simulink model "MyModel_Open_v1_r2016b"  (R2016b)
settings: Solver=ode23tb  StartTime=0.0  StopTime=0.3  MaxStep=1e-6  RelTol=1e-4
InitFcn:
  | Udc1 = 200;
  | Udc2 = 200;
  | tpwm = 1e-4;
  | ratio = Udc1/Udc2;
  | Td = 2e-6;
  | Kp_current = 3;
  | Ki_current = 120;
libraries: powerlib x31, powerlib_meascontrol x24, powerlib_extras x5, simulink_extras x2, simulink x2
(part 1 of 2)
settings Model: Creator=chenhao  LastModifiedBy=chenhao
settings SFSimCC: SimUseLocalCustomCode=on
settings RTWCC: RTWUseLocalCustomCode=on

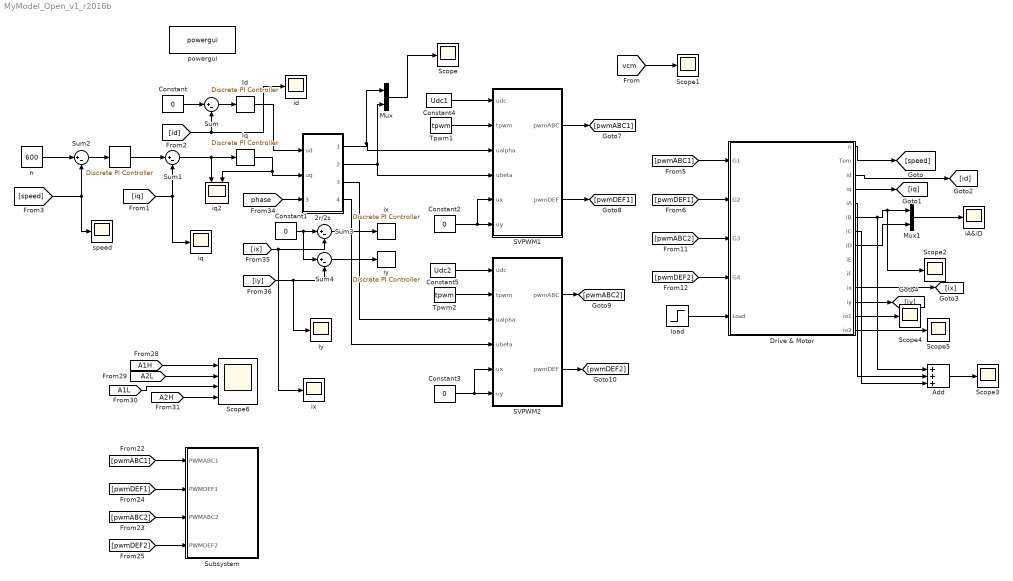
== system MyModel_Open_v1_r2016b ==
  "    " : powerlib_extras/Discrete  Control Blocks/Discrete PI Controller  Kp=1  Ki=100  Par_Limits=[50 -50]  Init=0  Ts=tpwm
  " Id" : powerlib_extras/Discrete  Control Blocks/Discrete PI Controller  Kp=Kp_current  Ki=Ki_current  Par_Limits=[300 -300]  Init=0  Ts=tpwm
  " Iq" : powerlib_extras/Discrete  Control Blocks/Discrete PI Controller  Kp=Kp_current  Ki=Ki_current  Par_Limits=[300 -300]  Init=0  Ts=tpwm
  " ix" : powerlib_extras/Discrete  Control Blocks/Discrete PI Controller  Kp=10  Ki=100  Par_Limits=[300 -300]  Init=0  Ts=tpwm
  " iy" : powerlib_extras/Discrete  Control Blocks/Discrete PI Controller  Kp=10  Ki=100  Par_Limits=[300 -300]  Init=0  Ts=tpwm
  2r/2s : Subsystem
  Add : Sum  Inputs=3
  Constant{,1..3} (4 alike) : Constant  Value=0
  Constant4 : Constant  Value=Udc1
  Constant5 : Constant  Value=Udc2
  Drive & Motor : Subsystem
  Mux : Mux  Inputs=2
  Mux1 : Mux  Inputs=2
  SVPWM1 : Subsystem
  SVPWM2 : Subsystem
  Scope{,1..5} (6 alike) : Scope
  Scope6 : Scope  NumInputPorts=4
  Subsystem : Subsystem
  Sum{,1..4} (5 alike) : Sum  Inputs=|+-
  Tpwm1 : Constant  Value=tpwm
  Tpwm2 : Constant  Value=tpwm
  "iA&iD " : Scope
  "id " : Scope
  iq : Scope
  iq2 : Scope  NumInputPorts=2
  ix : Scope
  iy : Scope
  load : Step  Time=0  After=15  SampleTime=0
  n : Constant  Value=600
  powergui : powerlib/powergui  Priority=1  SimulationMode=Continuous  SampleTime=1E-6  frequency=60  Iterations=50  frequencyindice=0  Pbase=100e6  ErrMax=1e-4  UnitsV=kV  UnitsW=MW  buscounter=0  FunctionMessages=off  echomessages=off  EnableUseOfTLC=off  CurrentSourceSwitches=off  DisableSnubberDevices=off  DisableRonSwitches=off  DisableVfSwitches=off  DisplayEquations=off  SolverType=Tustin/Backward Euler (TBE)  Interpol=off  ExternalGateDelay=off  methode=off  Ts=100  x0status=blocks  SPID=off  SwTol=0  HookPort=off  RestoreLinks=warning  ResistiveCurrentMeasurement=off  Frange=[0:2:500]  Ylog=off  Xlog=on  ShowGrid=off  save=off  variable=ZData  structure=IA  ZoomFFT=off  StartTime=0.2  cycles=3  DisplayStyle=1  fundamental=50  FreqAxis=on  MaxFrequency=1000  frequencyindicesteady=1  RmsSteady=1  display=off
  "speed " : Scope
  wires:
  2r/2s/2(ubeta1) -> SVPWM1/4(ubeta), Mux/2
  Mux/1 -> Scope/1
  Tpwm1/1 -> SVPWM1/2(tpwm)
  load/1 -> Drive & Motor/5(Load)
  [iy] -> iy/1, Sum4/2
  [iq] -> iq/1, Sum1/2
  Sum3/1 -> " ix"/1
  Constant4/1 -> SVPWM1/1(udc)
  Sum2/1 -> "    "/1
  2r/2s/1(ualfa1) -> SVPWM1/3(ualpha), Mux/1
  Sum1/1 -> iq2/1, " Iq"/1
  [speed] -> "speed "/1, Sum2/2
  Sum4/1 -> " iy"/1
  n/1 -> Sum2/1
  [ix] -> ix/1, Sum3/2
  " Id"/1 -> 2r/2s/1(ud)
  [phase] -> 2r/2s/3(theta)
  " Iq"/1 -> iq2/2, 2r/2s/2(uq)
  Sum/1 -> " Id"/1
  Constant1/1 -> Sum4/1, Sum3/1
  "    "/1 -> Sum1/1
  [id] -> "id "/1, Sum/2
  Constant/1 -> Sum/1
  Drive & Motor/1(n) -> [speed]
  Drive & Motor/4(iq) -> [iq]
  Drive & Motor/3(id) -> [id]
  Drive & Motor/11(ix) -> [ix]
  Drive & Motor/12(iy) -> [iy]
  Drive & Motor/5(iA) -> Add/1, Scope2/1, Mux1/1
  Drive & Motor/8(iD) -> Mux1/2
  Mux1/1 -> "iA&iD "/1
  Constant5/1 -> SVPWM2/1(udc)
  Tpwm2/1 -> SVPWM2/2(tpwm)
  2r/2s/3(ualfa2) -> SVPWM2/3(ualpha)
  2r/2s/4(ubeta2) -> SVPWM2/4(ubeta)
  Constant2/1 -> SVPWM1/5(ux), SVPWM1/6(uy)
  Constant3/1 -> SVPWM2/6(uy), SVPWM2/5(ux)
  SVPWM1/2(pwmDEF) -> [pwmDEF1]
  SVPWM2/1(pwmABC) -> [pwmABC2]
  SVPWM1/1(pwmABC) -> [pwmABC1]
  SVPWM2/2(pwmDEF) -> [pwmDEF2]
  [pwmABC1] -> Drive & Motor/1(G1)
  [pwmDEF1] -> Drive & Motor/2(G2)
  [pwmABC2] -> Drive & Motor/3(G3)
  [pwmDEF2] -> Drive & Motor/4(G4)
  [vcm] -> Scope1/1
  [A1L] -> Scope6/3
  [A1H] -> Scope6/1
  [pwmABC1] -> Subsystem/1(PWMABC1)
  [A2L] -> Scope6/2
  [A2H] -> Scope6/4
  [pwmDEF1] -> Subsystem/2(PWMDEF1)
  [pwmABC2] -> Subsystem/3(PWMABC2)
  [pwmDEF2] -> Subsystem/4(PWMDEF2)
  Drive & Motor/6(iB) -> Add/2
  Drive & Motor/7(iC) -> Add/3
  Add/1 -> Scope3/1
  Drive & Motor/13(io1) -> Scope4/1
  Drive & Motor/14(io2) -> Scope5/1

== system MyModel_Open_v1_r2016b/2r//2s ==
  ud : Inport
  uq : Inport  Port=2
  theta : Inport  Port=3
  Fcn : Fcn  Expr=u(1)*cos(u(3))-u(2)*sin(u(3))
  Fcn1 : Fcn  Expr=u(1)*sin(u(3))+u(2)*cos(u(3))
  Gain : Gain  Gain=ratio /(ratio + 1)
  Gain1 : Gain  Gain=ratio /(ratio + 1)
  Gain2 : Gain  Gain=-1 /(ratio + 1)
  Gain3 : Gain  Gain=-1 /(ratio + 1)
  Mux1 : Mux  Inputs=3
  ualfa1 : Outport
  ubeta1 : Outport  Port=2
  ualfa2 : Outport  Port=3
  ubeta2 : Outport  Port=4
  wires:
  theta/1 -> Mux1/3
  uq/1 -> Mux1/2
  ud/1 -> Mux1/1
  Mux1/1 -> Fcn1/1, Fcn/1
  Fcn/1 -> Gain2/1, Gain/1
  Gain/1 -> ualfa1/1
  Gain1/1 -> ubeta1/1
  Fcn1/1 -> Gain3/1, Gain1/1
  Gain2/1 -> ualfa2/1
  Gain3/1 -> ubeta2/1

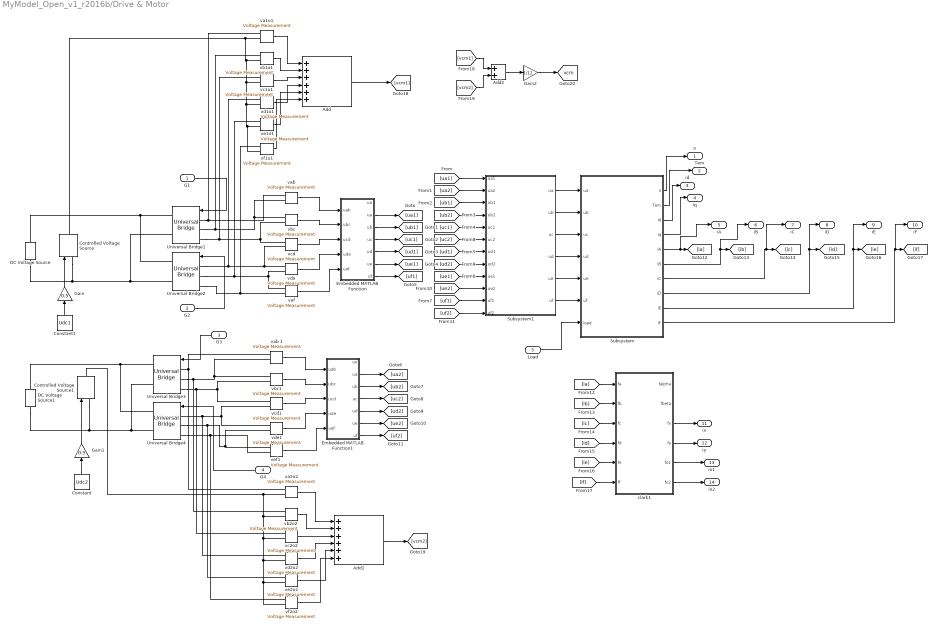
== system MyModel_Open_v1_r2016b/Drive & Motor ==
  G1 : Inport
  G2 : Inport  Port=2
  G3 : Inport  Port=3
  G4 : Inport  Port=4
  Load : Inport  Port=5
  Add : Sum  Inputs=++++++
  Add1 : Sum  Inputs=++++++
  Add2 : Sum
  Constant : Constant  Value=Udc2
  Constant1 : Constant  Value=Udc1
  Controlled Voltage Source : powerlib/Electrical Sources/Controlled Voltage Source  Initialize=on  Source_Type=AC  Amplitude=0  Phase=0  Frequency=0  Measurements=None
  Controlled Voltage Source1 : powerlib/Electrical Sources/Controlled Voltage Source  Initialize=on  Source_Type=AC  Amplitude=0  Phase=0  Frequency=0  Measurements=None
  DC Voltage Source : powerlib/Electrical Sources/DC Voltage Source  Amplitude=Udc1  Measurements=Voltage
  DC Voltage Source1 : powerlib/Electrical Sources/DC Voltage Source  Amplitude=Udc2  Measurements=Voltage
  Embedded MATLAB Function : MATLAB Function  TreatAsAtomicUnit=on
  Embedded MATLAB Function1 : MATLAB Function  TreatAsAtomicUnit=on
  Gain : Gain  Gain=0.5
  Gain1 : Gain  Gain=0.5
  Gain2 : Gain  Gain=1/12
  Subsystem : Subsystem
  Subsystem1 : Subsystem
  Universal Bridge{1..4} (4 alike) : powerlib/Power Electronics/Universal Bridge  Arms=3  SnubberResistance=1e5  SnubberCapacitance=inf  Device=IGBT / Diodes  Ron=1e-3  Lon=0  ForwardVoltages="[  0  0  ]"  ForwardVoltage=0  GTOparameters=[ 10e-6 , 20e-6 ]  IGBTparameters=[ 0 , 0 ]  Measurements=None  Measurements_2=None  converterType=Rectifier
  clark1 : MATLAB Function  TreatAsAtomicUnit=on
  va1o1 : powerlib/Measurements/Voltage Measurement  PhasorSimulation=off  OutputType=Complex  PSBequivalent=0
  va2o2 : powerlib/Measurements/Voltage Measurement  PhasorSimulation=off  OutputType=Complex  PSBequivalent=0
  "vab " : powerlib/Measurements/Voltage Measurement  PhasorSimulation=off  OutputType=Complex  PSBequivalent=0
  vab 1 : powerlib/Measurements/Voltage Measurement  PhasorSimulation=off  OutputType=Complex  PSBequivalent=0
  vb1o1 : powerlib/Measurements/Voltage Measurement  PhasorSimulation=off  OutputType=Complex  PSBequivalent=0
  vb2o2 : powerlib/Measurements/Voltage Measurement  PhasorSimulation=off  OutputType=Complex  PSBequivalent=0
  vbc : powerlib/Measurements/Voltage Measurement  PhasorSimulation=off  OutputType=Complex  PSBequivalent=0
  vbc1 : powerlib/Measurements/Voltage Measurement  PhasorSimulation=off  OutputType=Complex  PSBequivalent=0
  vc1o1 : powerlib/Measurements/Voltage Measurement  PhasorSimulation=off  OutputType=Complex  PSBequivalent=0
  vc2o2 : powerlib/Measurements/Voltage Measurement  PhasorSimulation=off  OutputType=Complex  PSBequivalent=0
  vcd : powerlib/Measurements/Voltage Measurement  PhasorSimulation=off  OutputType=Complex  PSBequivalent=0
  vcd1 : powerlib/Measurements/Voltage Measurement  PhasorSimulation=off  OutputType=Complex  PSBequivalent=0
  vd1o1 : powerlib/Measurements/Voltage Measurement  PhasorSimulation=off  OutputType=Complex  PSBequivalent=0
  vd2o2 : powerlib/Measurements/Voltage Measurement  PhasorSimulation=off  OutputType=Complex  PSBequivalent=0
  vde : powerlib/Measurements/Voltage Measurement  PhasorSimulation=off  OutputType=Complex  PSBequivalent=0
  vde1 : powerlib/Measurements/Voltage Measurement  PhasorSimulation=off  OutputType=Complex  PSBequivalent=0
  ve1o1 : powerlib/Measurements/Voltage Measurement  PhasorSimulation=off  OutputType=Complex  PSBequivalent=0
  ve2o2 : powerlib/Measurements/Voltage Measurement  PhasorSimulation=off  OutputType=Complex  PSBequivalent=0
  vef : powerlib/Measurements/Voltage Measurement  PhasorSimulation=off  OutputType=Complex  PSBequivalent=0
  vef1 : powerlib/Measurements/Voltage Measurement  PhasorSimulation=off  OutputType=Complex  PSBequivalent=0
  vf1o1 : powerlib/Measurements/Voltage Measurement  PhasorSimulation=off  OutputType=Complex  PSBequivalent=0
  vf2o2 : powerlib/Measurements/Voltage Measurement  PhasorSimulation=off  OutputType=Complex  PSBequivalent=0
  n : Outport
  Tem : Outport  Port=2
  id : Outport  Port=3
  iq : Outport  Port=4
  iA : Outport  Port=5
  iB : Outport  Port=6
  iC : Outport  Port=7
  iD : Outport  Port=8
  iE : Outport  Port=9
  iF : Outport  Port=10
  ix : Outport  Port=11
  iy : Outport  Port=12
  io1 : Outport  Port=13
  io2 : Outport  Port=14
  tag scope: vcm=global
  wires:
  G1/1 -> Universal Bridge1/1
  G2/1 -> Universal Bridge2/1
  G3/1 -> Universal Bridge3/1
  G4/1 -> Universal Bridge4/1
  vef/1 -> Embedded MATLAB Function/5(uef)
  vde/1 -> Embedded MATLAB Function/4(ude)
  "vab "/1 -> Embedded MATLAB Function/1(uab)
  vcd/1 -> Embedded MATLAB Function/3(ucd)
  vbc/1 -> Embedded MATLAB Function/2(ubc)
  Embedded MATLAB Function/2(ua) -> [ua1]
  Embedded MATLAB Function/3(ub) -> [ub1]
  Embedded MATLAB Function/4(uc) -> [uc1]
  Embedded MATLAB Function/5(ud) -> [ud1]
  Embedded MATLAB Function/6(ue) -> [ue1]
  Embedded MATLAB Function/7(uf) -> [uf1]
  Embedded MATLAB Function1/2(ua) -> [ua2]
  Embedded MATLAB Function1/3(ub) -> [ub2]
  Embedded MATLAB Function1/4(uc) -> [uc2]
  Embedded MATLAB Function1/5(ud) -> [ud2]
  Embedded MATLAB Function1/6(ue) -> [ue2]
  Embedded MATLAB Function1/7(uf) -> [uf2]
  vab 1/1 -> Embedded MATLAB Function1/1(uab)
  vbc1/1 -> Embedded MATLAB Function1/2(ubc)
  vcd1/1 -> Embedded MATLAB Function1/3(ucd)
  vde1/1 -> Embedded MATLAB Function1/4(ude)
  vef1/1 -> Embedded MATLAB Function1/5(uef)
  [ua1] -> Subsystem1/1(ua1)
  [ua2] -> Subsystem1/2(ua2)
  [ub1] -> Subsystem1/3(ub1)
  [ub2] -> Subsystem1/4(ub2)
  [uc1] -> Subsystem1/5(uc1)
  [uc2] -> Subsystem1/6(uc2)
  [ud1] -> Subsystem1/7(ud1)
  [ud2] -> Subsystem1/8(ud2)
  [ue1] -> Subsystem1/9(ue1)
  [ue2] -> Subsystem1/10(ue2)
  [uf1] -> Subsystem1/11(uf1)
  [uf2] -> Subsystem1/12(uf2)
  Subsystem1/1(ua) -> Subsystem/1(ua)
  Subsystem1/2(ub) -> Subsystem/2(ub)
  Subsystem1/3(uc) -> Subsystem/3(uc)
  Subsystem1/4(ud) -> Subsystem/4(ud)
  Subsystem1/5(ue) -> Subsystem/5(ue)
  Subsystem1/6(uf) -> Subsystem/6(uf)
  Load/1 -> Subsystem/7(load)
  Subsystem/1(n) -> n/1
  Subsystem/2(Tem) -> Tem/1
  Subsystem/3(id) -> id/1
  Subsystem/4(iq) -> iq/1
  Subsystem/5(iA) -> iA/1, [ia]
  Subsystem/6(iB) -> iB/1, [ib]
  Subsystem/7(iC) -> iC/1, [ic]
  Subsystem/8(iD) -> iD/1, [id]
  Subsystem/9(iE) -> iE/1, [ie]
  Subsystem/10(iF) -> iF/1, [if]
  [ia] -> clark1/1(fa)
  [ib] -> clark1/2(fb)
  [ic] -> clark1/3(fc)
  [id] -> clark1/4(fd)
  [ie] -> clark1/5(fe)
  [if] -> clark1/6(ff)
  clark1/3(fx) -> ix/1
  clark1/4(fy) -> iy/1
  Gain/1 -> Controlled Voltage Source/1
  Gain1/1 -> Controlled Voltage Source1/1
  va1o1/1 -> Add/1
  vb1o1/1 -> Add/2
  vc1o1/1 -> Add/3
  vd1o1/1 -> Add/4
  ve1o1/1 -> Add/5
  vf1o1/1 -> Add/6
  Add/1 -> [vcm1]
  va2o2/1 -> Add1/1
  vb2o2/1 -> Add1/2
  vc2o2/1 -> Add1/3
  vd2o2/1 -> Add1/4
  ve2o2/1 -> Add1/5
  vf2o2/1 -> Add1/6
  Add1/1 -> [vcm2]
  [vcm1] -> Add2/1
  [vcm2] -> Add2/2
  Add2/1 -> Gain2/1
  Gain2/1 -> [vcm]
  Constant/1 -> Gain1/1
  Constant1/1 -> Gain/1
  clark1/5(fo1) -> io1/1
  clark1/6(fo2) -> io2/1
  connections:
  vde1/LConn1 -- vcd1/LConn2 -- vd2o2/LConn1 -- Universal Bridge4/LConn1
  vde/LConn1 -- vd1o1/LConn1 -- Universal Bridge2/LConn1 -- vcd/LConn2
  vef1/LConn2 -- Universal Bridge4/LConn3 -- vf2o2/LConn1
  Universal Bridge1/RConn2 -- DC Voltage Source/LConn1 -- Controlled Voltage Source/LConn1 -- Universal Bridge2/RConn2
  DC Voltage Source/RConn1 -- Universal Bridge2/RConn1 -- Universal Bridge1/RConn1
  Universal Bridge3/LConn1 -- vab 1/LConn1 -- va2o2/LConn1
  vbc/LConn1 -- vb1o1/LConn1 -- Universal Bridge1/LConn2 -- "vab "/LConn2
  vbc1/LConn1 -- vb2o2/LConn1 -- Universal Bridge3/LConn2 -- vab 1/LConn2
  vcd/LConn1 -- vc1o1/LConn1 -- Universal Bridge1/LConn3 -- vbc/LConn2
  vbc1/LConn2 -- vc2o2/LConn1 -- Universal Bridge3/LConn3 -- vcd1/LConn1
  Universal Bridge3/RConn1 -- DC Voltage Source1/RConn1 -- Universal Bridge4/RConn1
  Universal Bridge3/RConn2 -- DC Voltage Source1/LConn1 -- Controlled Voltage Source1/LConn1 -- Universal Bridge4/RConn2
  vef1/LConn1 -- ve2o2/LConn1 -- Universal Bridge4/LConn2 -- vde1/LConn2
  Universal Bridge1/LConn1 -- "vab "/LConn1 -- va1o1/LConn1
  vef/LConn1 -- ve1o1/LConn1 -- Universal Bridge2/LConn2 -- vde/LConn2
  Universal Bridge2/LConn3 -- vf1o1/LConn1 -- vef/LConn2
  va1o1/LConn2 -- vf1o1/LConn2 -- ve1o1/LConn2 -- vd1o1/LConn2 -- vc1o1/LConn2 -- vb1o1/LConn2 -- Controlled Voltage Source/RConn1
  va2o2/LConn2 -- vf2o2/LConn2 -- ve2o2/LConn2 -- vd2o2/LConn2 -- vc2o2/LConn2 -- vb2o2/LConn2 -- Controlled Voltage Source1/RConn1

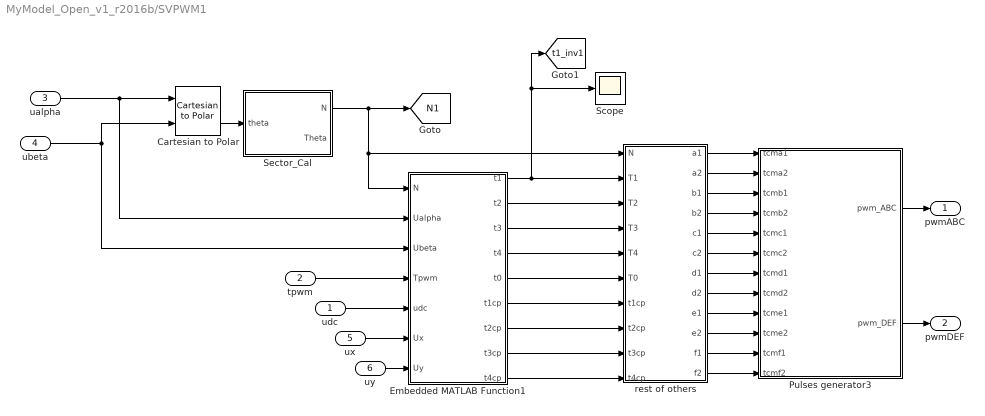
== system MyModel_Open_v1_r2016b/SVPWM1 ==
  udc : Inport
  tpwm : Inport  Port=2
  ualpha : Inport  Port=3
  ubeta : Inport  Port=4
  ux : Inport  Port=5
  uy : Inport  Port=6
  Cartesian to Polar : simulink_extras/Transformations/Cartesian to Polar
  Embedded MATLAB Function1 : MATLAB Function  TreatAsAtomicUnit=on
  Pulses generator3 : Subsystem
  Scope : Scope
  Sector_Cal : Subsystem
  rest of others : MATLAB Function  TreatAsAtomicUnit=on
  pwmABC : Outport
  pwmDEF : Outport  Port=2
  tag scope: N1=global, t1_inv1=global
  wires:
  tpwm/1 -> Embedded MATLAB Function1/4(Tpwm)
  ubeta/1 -> Cartesian to Polar/2, Embedded MATLAB Function1/3(Ubeta)
  ualpha/1 -> Cartesian to Polar/1, Embedded MATLAB Function1/2(Ualpha)
  ux/1 -> Embedded MATLAB Function1/6(Ux)
  uy/1 -> Embedded MATLAB Function1/7(Uy)
  udc/1 -> Embedded MATLAB Function1/5(udc)
  rest of others/12(f2) -> Pulses generator3/12(tcmf2)
  rest of others/11(f1) -> Pulses generator3/11(tcmf1)
  rest of others/9(e1) -> Pulses generator3/9(tcme1)
  rest of others/8(d2) -> Pulses generator3/8(tcmd2)
  rest of others/10(e2) -> Pulses generator3/10(tcme2)
  rest of others/2(a2) -> Pulses generator3/2(tcma2)
  rest of others/6(c2) -> Pulses generator3/6(tcmc2)
  rest of others/4(b2) -> Pulses generator3/4(tcmb2)
  rest of others/5(c1) -> Pulses generator3/5(tcmc1)
  rest of others/7(d1) -> Pulses generator3/7(tcmd1)
  rest of others/3(b1) -> Pulses generator3/3(tcmb1)
  rest of others/1(a1) -> Pulses generator3/1(tcma1)
  Embedded MATLAB Function1/1(t1) -> [t1_inv1], Scope/1, rest of others/2(T1)
  Embedded MATLAB Function1/2(t2) -> rest of others/3(T2)
  Embedded MATLAB Function1/3(t3) -> rest of others/4(T3)
  Embedded MATLAB Function1/4(t4) -> rest of others/5(T4)
  Embedded MATLAB Function1/5(t0) -> rest of others/6(T0)
  Embedded MATLAB Function1/6(t1cp) -> rest of others/7(t1cp)
  Embedded MATLAB Function1/7(t2cp) -> rest of others/8(t2cp)
  Embedded MATLAB Function1/8(t3cp) -> rest of others/9(t3cp)
  Embedded MATLAB Function1/9(t4cp) -> rest of others/10(t4cp)
  Cartesian to Polar/2 -> Sector_Cal/1(theta)
  Sector_Cal/1(N) -> [N1], rest of others/1(N), Embedded MATLAB Function1/1(N)
  Pulses generator3/1(pwm_ABC) -> pwmABC/1
  Pulses generator3/2(pwm_DEF) -> pwmDEF/1

== system MyModel_Open_v1_r2016b/SVPWM2 ==
  udc : Inport
  tpwm : Inport  Port=2
  ualpha : Inport  Port=3
  ubeta : Inport  Port=4
  ux : Inport  Port=5
  uy : Inport  Port=6
  Cartesian to Polar : simulink_extras/Transformations/Cartesian to Polar
  Embedded MATLAB Function1 : MATLAB Function  TreatAsAtomicUnit=on
  Pulses generator3 : Subsystem
  Scope : Scope
  Sector_Cal : Subsystem
  rest of others : MATLAB Function  TreatAsAtomicUnit=on
  pwmABC : Outport
  pwmDEF : Outport  Port=2
  tag scope: N2=global, t1_inv2=global
  wires:
  Pulses generator3/2(pwm_DEF) -> pwmDEF/1
  Pulses generator3/1(pwm_ABC) -> pwmABC/1
  Sector_Cal/1(N) -> [N2], Embedded MATLAB Function1/1(N), rest of others/1(N)
  Cartesian to Polar/2 -> Sector_Cal/1(theta)
  Embedded MATLAB Function1/9(t4cp) -> rest of others/10(t4cp)
  Embedded MATLAB Function1/8(t3cp) -> rest of others/9(t3cp)
  Embedded MATLAB Function1/7(t2cp) -> rest of others/8(t2cp)
  Embedded MATLAB Function1/6(t1cp) -> rest of others/7(t1cp)
  Embedded MATLAB Function1/5(t0) -> rest of others/6(T0)
  Embedded MATLAB Function1/4(t4) -> rest of others/5(T4)
  Embedded MATLAB Function1/3(t3) -> rest of others/4(T3)
  Embedded MATLAB Function1/2(t2) -> rest of others/3(T2)
  Embedded MATLAB Function1/1(t1) -> rest of others/2(T1), [t1_inv2], Scope/1
  rest of others/1(a1) -> Pulses generator3/1(tcma1)
  rest of others/3(b1) -> Pulses generator3/3(tcmb1)
  rest of others/7(d1) -> Pulses generator3/7(tcmd1)
  rest of others/5(c1) -> Pulses generator3/5(tcmc1)
  rest of others/4(b2) -> Pulses generator3/4(tcmb2)
  rest of others/6(c2) -> Pulses generator3/6(tcmc2)
  rest of others/2(a2) -> Pulses generator3/2(tcma2)
  rest of others/10(e2) -> Pulses generator3/10(tcme2)
  rest of others/8(d2) -> Pulses generator3/8(tcmd2)
  rest of others/9(e1) -> Pulses generator3/9(tcme1)
  rest of others/11(f1) -> Pulses generator3/11(tcmf1)
  rest of others/12(f2) -> Pulses generator3/12(tcmf2)
  udc/1 -> Embedded MATLAB Function1/5(udc)
  uy/1 -> Embedded MATLAB Function1/7(Uy)
  ux/1 -> Embedded MATLAB Function1/6(Ux)
  ualpha/1 -> Embedded MATLAB Function1/2(Ualpha), Cartesian to Polar/1
  ubeta/1 -> Embedded MATLAB Function1/3(Ubeta), Cartesian to Polar/2
  tpwm/1 -> Embedded MATLAB Function1/4(Tpwm)

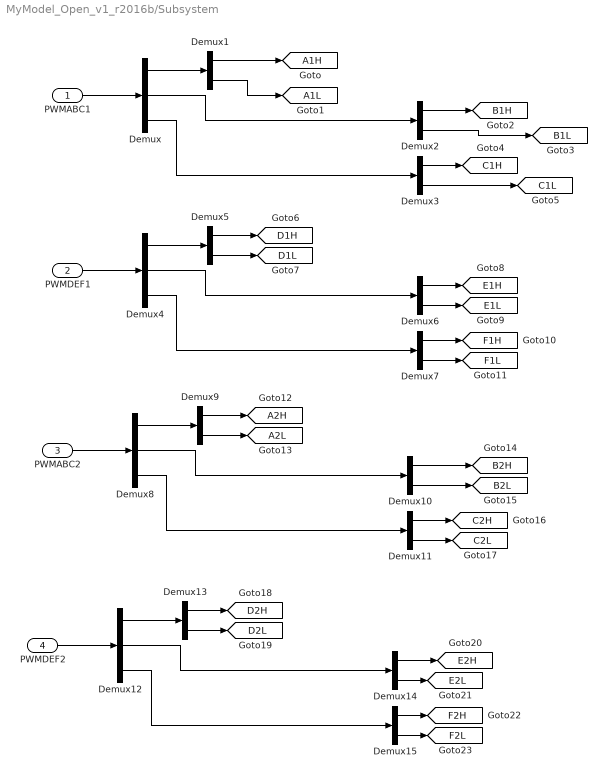
== system MyModel_Open_v1_r2016b/Subsystem ==
  PWMABC1 : Inport
  PWMDEF1 : Inport  Port=2
  PWMABC2 : Inport  Port=3
  PWMDEF2 : Inport  Port=4
  Demux{,4,8,12} (4 alike) : Demux  Outputs=3
  Demux{1..3,5..7,9..11,13..15} (12 alike) : Demux  Outputs=2
  tag scope: A1H=global, A1L=global, A2H=global, A2L=global, B1H=global, B1L=global, B2H=global, B2L=global, C1H=global, C1L=global, C2H=global, C2L=global, D1H=global, D1L=global, D2H=global, D2L=global, E1H=global, E1L=global, E2H=global, E2L=global, F1H=global, F1L=global, F2H=global, F2L=global
  wires:
  PWMABC1/1 -> Demux/1
  Demux/1 -> Demux1/1
  Demux/2 -> Demux2/1
  Demux/3 -> Demux3/1
  Demux4/3 -> Demux7/1
  Demux4/2 -> Demux6/1
  Demux4/1 -> Demux5/1
  PWMDEF1/1 -> Demux4/1
  PWMABC2/1 -> Demux8/1
  Demux8/1 -> Demux9/1
  Demux8/2 -> Demux10/1
  Demux8/3 -> Demux11/1
  Demux12/3 -> Demux15/1
  Demux12/2 -> Demux14/1
  Demux12/1 -> Demux13/1
  PWMDEF2/1 -> Demux12/1
  Demux1/1 -> [A1H]
  Demux1/2 -> [A1L]
  Demux2/1 -> [B1H]
  Demux2/2 -> [B1L]
  Demux3/1 -> [C1H]
  Demux3/2 -> [C1L]
  Demux5/1 -> [D1H]
  Demux5/2 -> [D1L]
  Demux6/1 -> [E1H]
  Demux6/2 -> [E1L]
  Demux7/1 -> [F1H]
  Demux7/2 -> [F1L]
  Demux9/1 -> [A2H]
  Demux9/2 -> [A2L]
  Demux10/1 -> [B2H]
  Demux10/2 -> [B2L]
  Demux11/1 -> [C2H]
  Demux11/2 -> [C2L]
  Demux13/1 -> [D2H]
  Demux13/2 -> [D2L]
  Demux14/1 -> [E2H]
  Demux14/2 -> [E2L]
  Demux15/1 -> [F2H]
  Demux15/2 -> [F2L]

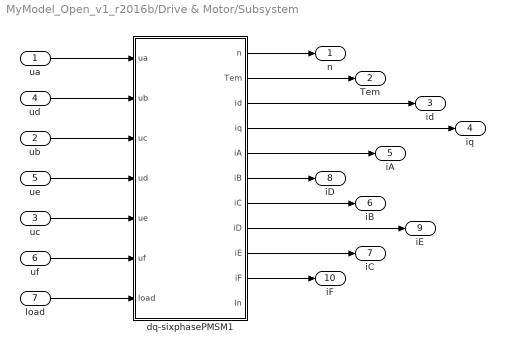
== system MyModel_Open_v1_r2016b/Drive & Motor/Subsystem ==
  ua : Inport
  ub : Inport  Port=2
  uc : Inport  Port=3
  ud : Inport  Port=4
  ue : Inport  Port=5
  uf : Inport  Port=6
  load : Inport  Port=7
  dq-sixphasePMSM1 : Subsystem  mask{R=0.099, Ld=2.463342136542000e-03, Lq=2.473254136542000e-03, Lf=1.520747e-3, psi=0.0592, p=5, J=0.00174}
      mask prompts: R "Resistance (Om)"; Ld "d-inductance (H)"; Lq "q-inductance (H)"; Lf "Leak inductance (H)"; psi "flux (Wb)"; p "pole pairs"; J "inertia (kg*m^2)"
  n : Outport
  Tem : Outport  Port=2
  id : Outport  Port=3
  iq : Outport  Port=4
  iA : Outport  Port=5
  iB : Outport  Port=6
  iC : Outport  Port=7
  iD : Outport  Port=8
  iE : Outport  Port=9
  iF : Outport  Port=10
  wires:
  dq-sixphasePMSM1/10(iF) -> iF/1
  dq-sixphasePMSM1/4(iq) -> iq/1
  ue/1 -> dq-sixphasePMSM1/4(ud)
  dq-sixphasePMSM1/8(iD) -> iE/1
  uf/1 -> dq-sixphasePMSM1/6(uf)
  dq-sixphasePMSM1/7(iC) -> iB/1
  dq-sixphasePMSM1/5(iA) -> iA/1
  dq-sixphasePMSM1/2(Tem) -> Tem/1
  ua/1 -> dq-sixphasePMSM1/1(ua)
  dq-sixphasePMSM1/3(id) -> id/1
  ud/1 -> dq-sixphasePMSM1/2(ub)
  dq-sixphasePMSM1/9(iE) -> iC/1
  dq-sixphasePMSM1/1(n) -> n/1
  load/1 -> dq-sixphasePMSM1/7(load)
  uc/1 -> dq-sixphasePMSM1/5(ue)
  dq-sixphasePMSM1/6(iB) -> iD/1
  ub/1 -> dq-sixphasePMSM1/3(uc)

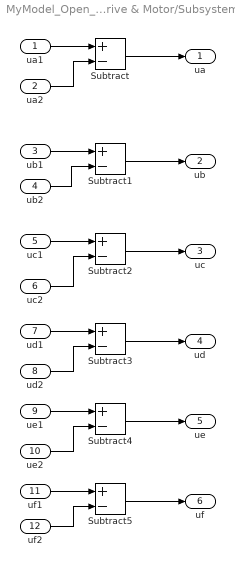
== system MyModel_Open_v1_r2016b/Drive & Motor/Subsystem1 ==
  ua1 : Inport
  ua2 : Inport  Port=2
  ub1 : Inport  Port=3
  ub2 : Inport  Port=4
  uc1 : Inport  Port=5
  uc2 : Inport  Port=6
  ud1 : Inport  Port=7
  ud2 : Inport  Port=8
  ue1 : Inport  Port=9
  ue2 : Inport  Port=10
  uf1 : Inport  Port=11
  uf2 : Inport  Port=12
  Subtract{,1..5} (6 alike) : Sum  Inputs=+-
  ua : Outport
  ub : Outport  Port=2
  uc : Outport  Port=3
  ud : Outport  Port=4
  ue : Outport  Port=5
  uf : Outport  Port=6
  wires:
  ua1/1 -> Subtract/1
  ua2/1 -> Subtract/2
  Subtract/1 -> ua/1
  ub1/1 -> Subtract1/1
  ub2/1 -> Subtract1/2
  Subtract1/1 -> ub/1
  uc1/1 -> Subtract2/1
  uc2/1 -> Subtract2/2
  Subtract2/1 -> uc/1
  ud1/1 -> Subtract3/1
  ud2/1 -> Subtract3/2
  Subtract3/1 -> ud/1
  ue1/1 -> Subtract4/1
  ue2/1 -> Subtract4/2
  Subtract4/1 -> ue/1
  uf1/1 -> Subtract5/1
  uf2/1 -> Subtract5/2
  Subtract5/1 -> uf/1

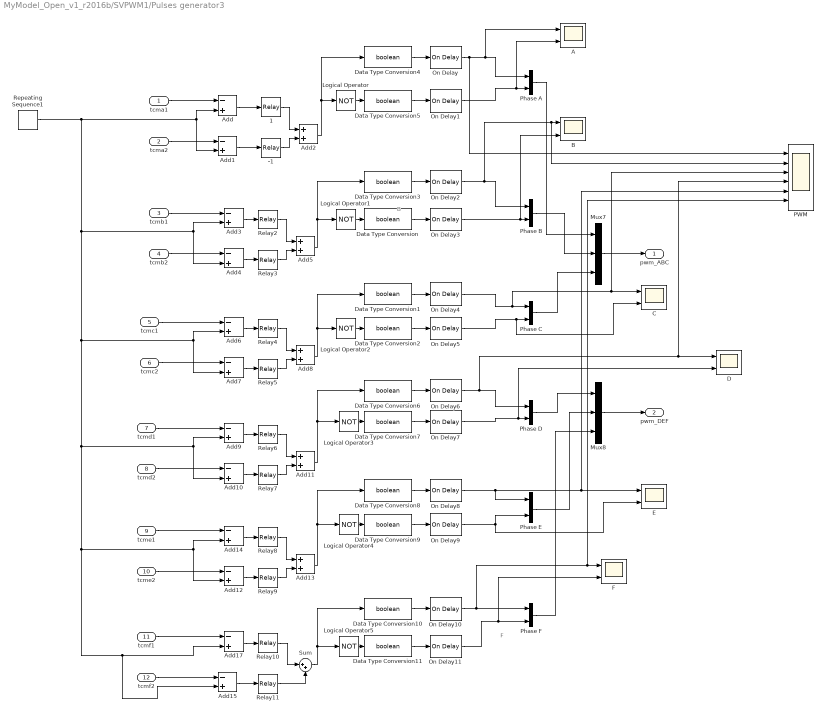
== system MyModel_Open_v1_r2016b/SVPWM1/Pulses generator3 ==
  note: B
  note: F
  tcma1 : Inport
  tcma2 : Inport  Port=2
  tcmb1 : Inport  Port=3
  tcmb2 : Inport  Port=4
  tcmc1 : Inport  Port=5
  tcmc2 : Inport  Port=6
  tcmd1 : Inport  Port=7
  tcmd2 : Inport  Port=8
  tcme1 : Inport  Port=9
  tcme2 : Inport  Port=10
  tcmf1 : Inport  Port=11
  tcmf2 : Inport  Port=12
  -1 : Relay  OnOutputValue=-1
  1 : Relay
  A : Scope  NumInputPorts=2
  Add{,1,3..4,6..7,9..10,12,14..15,17} (12 alike) : Sum  Inputs=-+
  Add{2,5,8,11,13} (5 alike) : Sum
  B : Scope  NumInputPorts=2
  C : Scope  NumInputPorts=2
  D : Scope  NumInputPorts=2
  Data Type Conversion{,1..11} (12 alike) : DataTypeConversion  OutDataTypeStr=boolean
  E : Scope  NumInputPorts=2
  F : Scope  NumInputPorts=2
  Logical Operator{,1..5} (6 alike) : Logic  Operator=NOT  AllPortsSameDT=off  OutDataTypeStr=boolean
  Mux7 : Mux  Inputs=3
  Mux8 : Mux  Inputs=3
  On Delay{,1..11} (12 alike) : powerlib_meascontrol/Logic/On Delay  DelayType=On delay  delay=Td  ic=0  Ts=0
  PWM : Scope  NumInputPorts=6
  Phase A : Mux  Inputs=2
  Phase B : Mux  Inputs=2
  Phase C : Mux  Inputs=2
  Phase D : Mux  Inputs=2
  Phase E : Mux  Inputs=2
  Phase F : Mux  Inputs=2
  Relay{2,4,6,8,10} (5 alike) : Relay
  Relay{3,5,7,9,11} (5 alike) : Relay  OnOutputValue=-1
  Repeating Sequence1 : simulink/Sources/Repeating Sequence  rep_seq_t=[0 tpwm]  rep_seq_y=[0 tpwm]
  Sum : Sum  Inputs=|++
  pwm_ABC : Outport
  pwm_DEF : Outport  Port=2
  wires:
  On Delay11/1 -> F/2, Phase F/2
  Data Type Conversion11/1 -> On Delay11/1
  On Delay10/1 -> PWM/6, F/1, Phase F/1
  Data Type Conversion10/1 -> On Delay10/1
  On Delay9/1 -> E/2, Phase E/2
  Data Type Conversion9/1 -> On Delay9/1
  On Delay8/1 -> Phase E/1, PWM/5, E/1
  Data Type Conversion8/1 -> On Delay8/1
  On Delay7/1 -> D/2, Phase D/2
  Data Type Conversion7/1 -> On Delay7/1
  On Delay6/1 -> PWM/4, D/1, Phase D/1
  Data Type Conversion6/1 -> On Delay6/1
  On Delay5/1 -> C/2, Phase C/2
  Data Type Conversion2/1 -> On Delay5/1
  On Delay4/1 -> PWM/3, C/1, Phase C/1
  Data Type Conversion1/1 -> On Delay4/1
  On Delay2/1 -> PWM/2, B/1, Phase B/1
  On Delay3/1 -> B/2, Phase B/2
  Data Type Conversion/1 -> On Delay3/1
  Data Type Conversion3/1 -> On Delay2/1
  On Delay1/1 -> A/2, Phase A/2
  Data Type Conversion5/1 -> On Delay1/1
  On Delay/1 -> A/1, Phase A/1, PWM/1
  Data Type Conversion4/1 -> On Delay/1
  Logical Operator3/1 -> Data Type Conversion7/1
  Logical Operator2/1 -> Data Type Conversion2/1
  Logical Operator/1 -> Data Type Conversion5/1
  Logical Operator1/1 -> Data Type Conversion/1
  Logical Operator4/1 -> Data Type Conversion9/1
  Add5/1 -> Logical Operator1/1, Data Type Conversion3/1
  Add2/1 -> Logical Operator/1, Data Type Conversion4/1
  Mux8/1 -> pwm_DEF/1
  Mux7/1 -> pwm_ABC/1
  Sum/1 -> Data Type Conversion10/1, Logical Operator5/1
  Add13/1 -> Data Type Conversion8/1, Logical Operator4/1
  Add11/1 -> Data Type Conversion6/1, Logical Operator3/1
  Add8/1 -> Data Type Conversion1/1, Logical Operator2/1
  Logical Operator5/1 -> Data Type Conversion11/1
  tcmf2/1 -> Add15/1
  Relay11/1 -> Sum/2
  Relay10/1 -> Sum/1
  Add17/1 -> Relay10/1
  tcmf1/1 -> Add17/1
  tcme2/1 -> Add12/1
  Relay9/1 -> Add13/2
  Relay8/1 -> Add13/1
  Add12/1 -> Relay9/1
  Add14/1 -> Relay8/1
  tcme1/1 -> Add14/1
  tcmd2/1 -> Add10/1
  Relay7/1 -> Add11/2
  Relay6/1 -> Add11/1
  Add10/1 -> Relay7/1
  Add9/1 -> Relay6/1
  tcmd1/1 -> Add9/1
  tcmc2/1 -> Add7/1
  Relay5/1 -> Add8/2
  Relay4/1 -> Add8/1
  Add7/1 -> Relay5/1
  Add6/1 -> Relay4/1
  tcmb2/1 -> Add4/1
  Relay3/1 -> Add5/2
  Relay2/1 -> Add5/1
  Add4/1 -> Relay3/1
  Add3/1 -> Relay2/1
  tcma1/1 -> Add/1
  -1/1 -> Add2/2
  1/1 -> Add2/1
  Add1/1 -> -1/1
  Add/1 -> 1/1
  Repeating Sequence1/1 -> Add15/2, Add17/2, Add12/2, Add14/2, Add9/2, Add10/2, Add7/2, Add6/2, Add3/2, Add4/2, Add1/2, Add/2
  tcma2/1 -> Add1/1
  tcmb1/1 -> Add3/1
  tcmc1/1 -> Add6/1
  Add15/1 -> Relay11/1
  Phase A/1 -> Mux7/1
  Phase B/1 -> Mux7/2
  Phase C/1 -> Mux7/3
  Phase D/1 -> Mux8/1
  Phase E/1 -> Mux8/2
  Phase F/1 -> Mux8/3

== system MyModel_Open_v1_r2016b/SVPWM1/Sector_Cal ==
  theta : Inport
  Add : Sum
  Constant : Constant  Value=pi/6
  Constant1 : Constant  Value=12
  Constant2 : Constant
  Constant3 : Constant  Value=pi/12
  Constant4 : Constant  Value=pi/6
  Divide : Product  Inputs=*/
  Math Function : Math  Operator=mod  SaturateOnIntegerOverflow=on
  Math Function1 : Math  Operator=mod  SaturateOnIntegerOverflow=on
  Rounding Function : Rounding
  Saturation : Saturate  UpperLimit=12  LowerLimit=1
  Sum : Sum  Inputs=|++
  N : Outport
  Theta : Outport  Port=2
  wires:
  Constant/1 -> Divide/2
  Divide/1 -> Rounding Function/1
  Rounding Function/1 -> Math Function/1
  Constant1/1 -> Math Function/2
  Math Function/1 -> Add/1
  Constant2/1 -> Add/2
  Add/1 -> Saturation/1
  Saturation/1 -> N/1
  theta/1 -> Sum/1
  Sum/1 -> Math Function1/1, Divide/1
  Constant3/1 -> Sum/2
  Constant4/1 -> Math Function1/2
  Math Function1/1 -> Theta/1

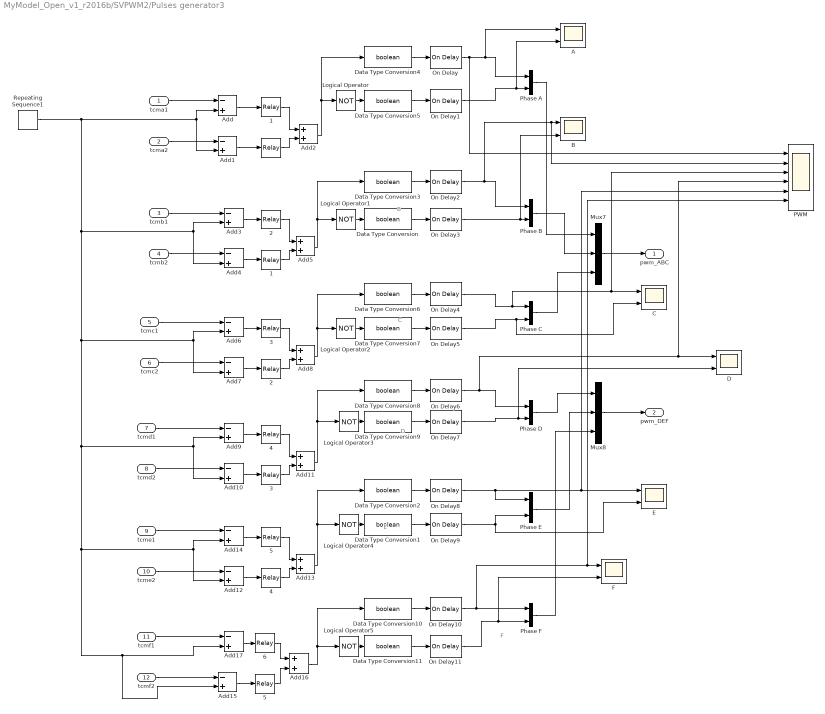
== system MyModel_Open_v1_r2016b/SVPWM2/Pulses generator3 ==
  note: F
  note: E
  note: D
  note: C
  note: B
  tcma1 : Inport
  tcma2 : Inport  Port=2
  tcmb1 : Inport  Port=3
  tcmb2 : Inport  Port=4
  tcmc1 : Inport  Port=5
  tcmc2 : Inport  Port=6
  tcmd1 : Inport  Port=7
  tcmd2 : Inport  Port=8
  tcme1 : Inport  Port=9
  tcme2 : Inport  Port=10
  tcmf1 : Inport  Port=11
  tcmf2 : Inport  Port=12
   {,1..5} (6 alike) : Relay
  {1..6} (6 alike) : Relay  OnOutputValue=0  OffOutputValue=1
  A : Scope  NumInputPorts=2
  Add{,1,3..4,6..7,9..10,12,14..15,17} (12 alike) : Sum  Inputs=-+
  Add{2,5,8,11,13,16} (6 alike) : Sum
  B : Scope  NumInputPorts=2
  C : Scope  NumInputPorts=2
  D : Scope  NumInputPorts=2
  Data Type Conversion{,1..11} (12 alike) : DataTypeConversion  OutDataTypeStr=boolean
  E : Scope  NumInputPorts=2
  F : Scope  NumInputPorts=2
  Logical Operator{,1..5} (6 alike) : Logic  Operator=NOT  AllPortsSameDT=off  OutDataTypeStr=boolean
  Mux7 : Mux  Inputs=3
  Mux8 : Mux  Inputs=3
  On Delay{,1..11} (12 alike) : powerlib_meascontrol/Logic/On Delay  DelayType=On delay  delay=Td  ic=0  Ts=0
  PWM : Scope  NumInputPorts=6
  Phase A : Mux  Inputs=2
  Phase B : Mux  Inputs=2
  Phase C : Mux  Inputs=2
  Phase D : Mux  Inputs=2
  Phase E : Mux  Inputs=2
  Phase F : Mux  Inputs=2
  Repeating Sequence1 : simulink/Sources/Repeating Sequence  rep_seq_t=[0 tpwm]  rep_seq_y=[0 tpwm]
  pwm_ABC : Outport
  pwm_DEF : Outport  Port=2
  wires:
  Phase F/1 -> Mux8/3
  Phase E/1 -> Mux8/2
  Phase D/1 -> Mux8/1
  Phase C/1 -> Mux7/3
  Phase B/1 -> Mux7/2
  Phase A/1 -> Mux7/1
  tcmc1/1 -> Add6/1
  tcmb1/1 -> Add3/1
  tcma2/1 -> Add1/1
  Repeating Sequence1/1 -> Add/2, Add1/2, Add4/2, Add3/2, Add6/2, Add7/2, Add10/2, Add9/2, Add14/2, Add12/2, Add17/2, Add15/2
  Add/1 -> 1/1
  Add1/1 -> " "/1
  1/1 -> Add2/1
  " "/1 -> Add2/2
  tcma1/1 -> Add/1
  tcmb2/1 -> Add4/1
  tcmc2/1 -> Add7/1
  tcmd1/1 -> Add9/1
  tcmd2/1 -> Add10/1
  tcme1/1 -> Add14/1
  tcme2/1 -> Add12/1
  tcmf1/1 -> Add17/1
  tcmf2/1 -> Add15/1
  Logical Operator5/1 -> Data Type Conversion11/1
  Add8/1 -> Data Type Conversion6/1, Logical Operator2/1
  Add11/1 -> Data Type Conversion8/1, Logical Operator3/1
  Add13/1 -> Data Type Conversion2/1, Logical Operator4/1
  Add16/1 -> Data Type Conversion10/1, Logical Operator5/1
  Mux7/1 -> pwm_ABC/1
  Mux8/1 -> pwm_DEF/1
  Add2/1 -> Data Type Conversion4/1, Logical Operator/1
  Add5/1 -> Data Type Conversion3/1, Logical Operator1/1
  Logical Operator4/1 -> Data Type Conversion1/1
  Logical Operator1/1 -> Data Type Conversion/1
  Logical Operator/1 -> Data Type Conversion5/1
  Logical Operator2/1 -> Data Type Conversion7/1
  Logical Operator3/1 -> Data Type Conversion9/1
  Data Type Conversion4/1 -> On Delay/1
  On Delay/1 -> PWM/1, Phase A/1, A/1
  Data Type Conversion5/1 -> On Delay1/1
  On Delay1/1 -> Phase A/2, A/2
  Data Type Conversion3/1 -> On Delay2/1
  Data Type Conversion/1 -> On Delay3/1
  On Delay3/1 -> Phase B/2, B/2
  On Delay2/1 -> Phase B/1, B/1, PWM/2
  Data Type Conversion6/1 -> On Delay4/1
  On Delay4/1 -> Phase C/1, C/1, PWM/3
  Data Type Conversion7/1 -> On Delay5/1
  On Delay5/1 -> Phase C/2, C/2
  Data Type Conversion8/1 -> On Delay6/1
  On Delay6/1 -> Phase D/1, D/1, PWM/4
  Data Type Conversion9/1 -> On Delay7/1
  On Delay7/1 -> Phase D/2, D/2
  Data Type Conversion2/1 -> On Delay8/1
  On Delay8/1 -> E/1, PWM/5, Phase E/1
  Data Type Conversion1/1 -> On Delay9/1
  On Delay9/1 -> Phase E/2, E/2
  Data Type Conversion10/1 -> On Delay10/1
  On Delay10/1 -> Phase F/1, F/1, PWM/6
  Data Type Conversion11/1 -> On Delay11/1
  On Delay11/1 -> Phase F/2, F/2
  " 1"/1 -> Add5/2
  2/1 -> Add5/1
  Add4/1 -> " 1"/1
  Add3/1 -> 2/1
  " 2"/1 -> Add8/2
  3/1 -> Add8/1
  Add7/1 -> " 2"/1
  Add6/1 -> 3/1
  4/1 -> Add11/1
  " 3"/1 -> Add11/2
  Add10/1 -> " 3"/1
  Add9/1 -> 4/1
  Add14/1 -> 5/1
  Add12/1 -> " 4"/1
  " 4"/1 -> Add13/2
  5/1 -> Add13/1
  6/1 -> Add16/1
  " 5"/1 -> Add16/2
  Add15/1 -> " 5"/1
  Add17/1 -> 6/1

== system MyModel_Open_v1_r2016b/SVPWM2/Sector_Cal ==
  theta : Inport
  Add : Sum
  Constant : Constant  Value=pi/6
  Constant1 : Constant  Value=12
  Constant2 : Constant
  Constant3 : Constant  Value=pi/12
  Constant4 : Constant  Value=pi/6
  Divide : Product  Inputs=*/
  Math Function : Math  Operator=mod  SaturateOnIntegerOverflow=on
  Math Function1 : Math  Operator=mod  SaturateOnIntegerOverflow=on
  Rounding Function : Rounding
  Saturation : Saturate  UpperLimit=12  LowerLimit=1
  Sum : Sum  Inputs=|++
  N : Outport
  Theta : Outport  Port=2
  wires:
  Math Function1/1 -> Theta/1
  Constant4/1 -> Math Function1/2
  Constant3/1 -> Sum/2
  Sum/1 -> Divide/1, Math Function1/1
  theta/1 -> Sum/1
  Saturation/1 -> N/1
  Add/1 -> Saturation/1
  Constant2/1 -> Add/2
  Math Function/1 -> Add/1
  Constant1/1 -> Math Function/2
  Rounding Function/1 -> Math Function/1
  Divide/1 -> Rounding Function/1
  Constant/1 -> Divide/2

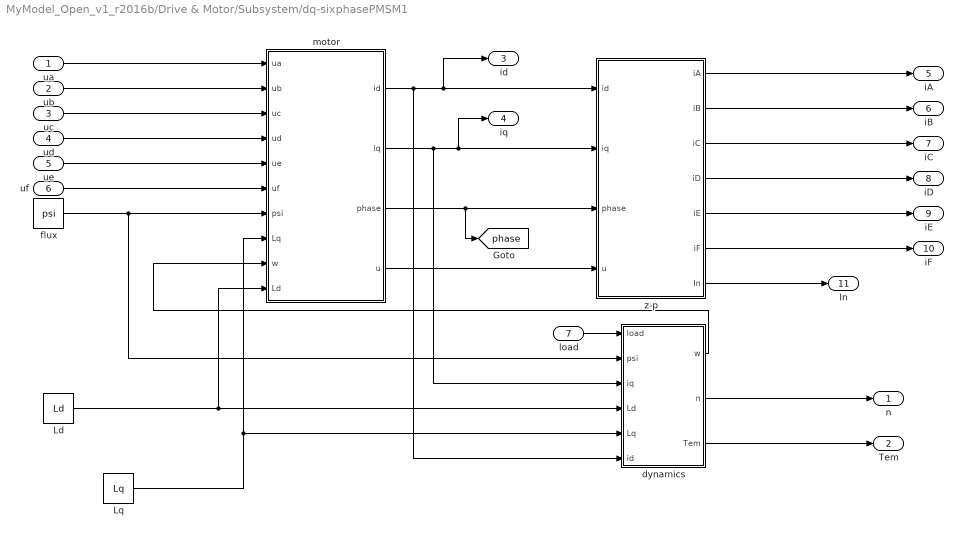
== system MyModel_Open_v1_r2016b/Drive & Motor/Subsystem/dq-sixphasePMSM1 ==
  ua : Inport
  ub : Inport  Port=2
  uc : Inport  Port=3
  ud : Inport  Port=4
  ue : Inport  Port=5
  uf : Inport  Port=6
  load : Inport  Port=7
  Ld : Constant  Value=Ld
  Lq : Constant  Value=Lq
  dynamics : Subsystem
  flux : Constant  Value=psi
  motor : Subsystem
  z-p : Subsystem
  n : Outport
  Tem : Outport  Port=2
  id : Outport  Port=3
  iq : Outport  Port=4
  iA : Outport  Port=5
  iB : Outport  Port=6
  iC : Outport  Port=7
  iD : Outport  Port=8
  iE : Outport  Port=9
  iF : Outport  Port=10
  In : Outport  Port=11
  tag scope: phase=global
  wires:
  Lq/1 -> motor/8(Lq), dynamics/5(Lq)
  Ld/1 -> dynamics/4(Ld), motor/10(Ld)
  ud/1 -> motor/4(ud)
  ua/1 -> motor/1(ua)
  ue/1 -> motor/5(ue)
  ub/1 -> motor/2(ub)
  uf/1 -> motor/6(uf)
  uc/1 -> motor/3(uc)
  dynamics/2(n) -> n/1
  load/1 -> dynamics/1(load)
  z-p/1(iA) -> iA/1
  motor/1(id) -> dynamics/6(id), z-p/1(id), id/1
  motor/2(iq) -> dynamics/3(iq), z-p/2(iq), iq/1
  motor/4(u) -> z-p/4(u)
  dynamics/1(w) -> motor/9(w)
  dynamics/3(Tem) -> Tem/1
  flux/1 -> dynamics/2(psi), motor/7(psi)
  z-p/2(iB) -> iB/1
  z-p/3(iC) -> iC/1
  z-p/4(iD) -> iD/1
  z-p/5(iE) -> iE/1
  z-p/6(iF) -> iF/1
  motor/3(phase) -> [phase], z-p/3(phase)
  z-p/7(In) -> In/1

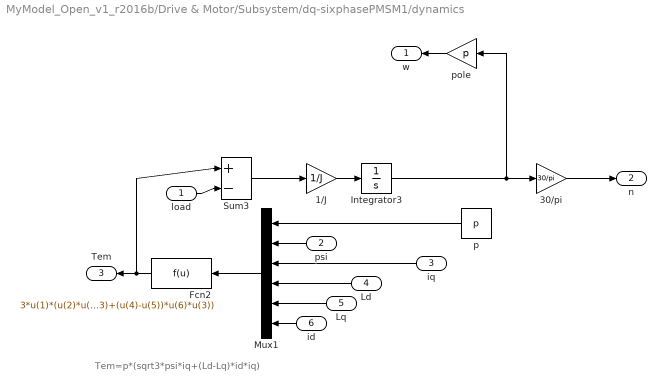
== system MyModel_Open_v1_r2016b/Drive & Motor/Subsystem/dq-sixphasePMSM1/dynamics ==
  note: Tem=p*(sqrt3*psi*iq+(Ld-Lq)*id*iq)
  load : Inport
  psi : Inport  Port=2
  iq : Inport  Port=3
  Ld : Inport  Port=4
  Lq : Inport  Port=5
  id : Inport  Port=6
  1/J : Gain  Gain=1/J  SaturateOnIntegerOverflow=on  OutDataTypeStr=Inherit: Same as input  ParamDataTypeStr=Inherit: Same as input
  30/pi : Gain  Gain=30/pi  SaturateOnIntegerOverflow=on  OutDataTypeStr=Inherit: Same as input  ParamDataTypeStr=Inherit: Same as input
  Fcn2 : Fcn  Expr=3*u(1)*(u(2)*u(3)+(u(4)-u(5))*u(6)*u(3))
  Integrator3 : Integrator
  Mux1 : Mux  Inputs=6
  Sum3 : Sum  Inputs=|+-  SaturateOnIntegerOverflow=on
  p : Constant  Value=p
  pole : Gain  Gain=p  SaturateOnIntegerOverflow=on  OutDataTypeStr=Inherit: Same as input  ParamDataTypeStr=Inherit: Same as input
  w : Outport
  n : Outport  Port=2
  Tem : Outport  Port=3
  wires:
  p/1 -> Mux1/1
  Mux1/1 -> Fcn2/1
  Fcn2/1 -> Sum3/1, Tem/1
  Sum3/1 -> 1/J/1
  1/J/1 -> Integrator3/1
  Integrator3/1 -> 30/pi/1, pole/1
  psi/1 -> Mux1/2
  Ld/1 -> Mux1/4
  Lq/1 -> Mux1/5
  pole/1 -> w/1
  30/pi/1 -> n/1
  load/1 -> Sum3/2
  iq/1 -> Mux1/3
  id/1 -> Mux1/6

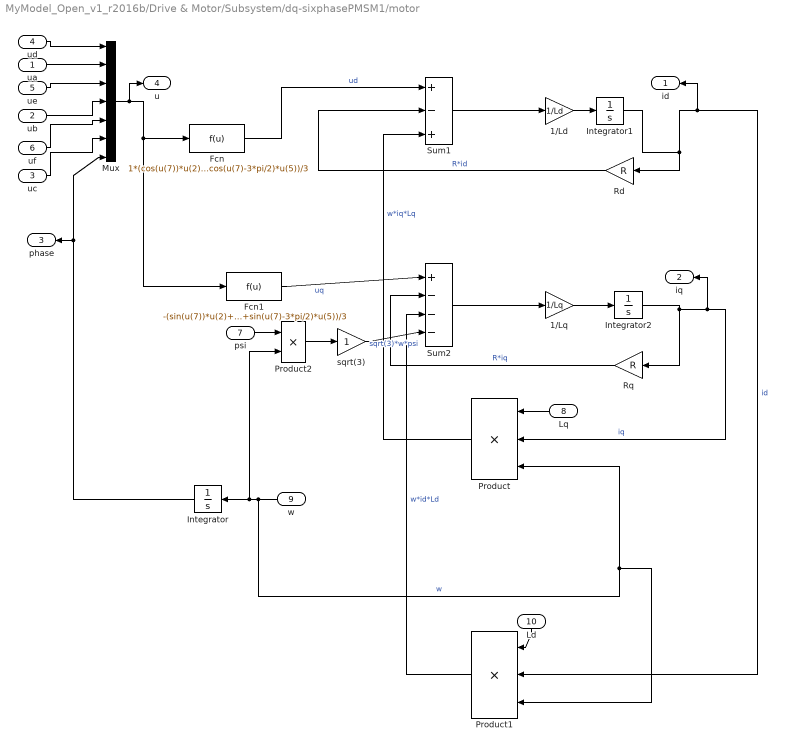
== system MyModel_Open_v1_r2016b/Drive & Motor/Subsystem/dq-sixphasePMSM1/motor ==
  ua : Inport
  ub : Inport  Port=2
  uc : Inport  Port=3
  ud : Inport  Port=4
  ue : Inport  Port=5
  uf : Inport  Port=6
  psi : Inport  Port=7
  Lq : Inport  Port=8
  w : Inport  Port=9
  Ld : Inport  Port=10
  1/Ld : Gain  Gain=1/Ld  SaturateOnIntegerOverflow=on  OutDataTypeStr=Inherit: Same as input  ParamDataTypeStr=Inherit: Same as input
  1/Lq : Gain  Gain=1/Lq  SaturateOnIntegerOverflow=on  OutDataTypeStr=Inherit: Same as input  ParamDataTypeStr=Inherit: Same as input
  Fcn : Fcn  Expr=1*(cos(u(7))*u(2)+cos(u(7)-pi/6)*u(4)+cos(u(7)-2*pi/3)*u(6)+cos(u(7)-5*pi/6)*u(1)+cos(u(7)-4*pi/3)*u(3)+cos(u(7)-3*pi/2)*u(5))/3
  Fcn1 : Fcn  Expr=-(sin(u(7))*u(2)+sin(u(7)-pi/6)*u(4)+sin(u(7)-2*pi/3)*u(6)+sin(u(7)-5*pi/6)*u(1)+sin(u(7)-4*pi/3)*u(3)+sin(u(7)-3*pi/2)*u(5))/3
  Integrator : Integrator
  Integrator1 : Integrator
  Integrator2 : Integrator
  Mux : Mux  Inputs=7
  Product : Product  Inputs=3  SaturateOnIntegerOverflow=on  OutDataTypeStr=Inherit: Same as first input
  Product1 : Product  Inputs=3  SaturateOnIntegerOverflow=on  OutDataTypeStr=Inherit: Same as first input
  Product2 : Product  SaturateOnIntegerOverflow=on  OutDataTypeStr=Inherit: Same as first input
  Rd : Gain  Gain=R  SaturateOnIntegerOverflow=on  OutDataTypeStr=Inherit: Same as input  ParamDataTypeStr=Inherit: Same as input
  Rq : Gain  Gain=R  SaturateOnIntegerOverflow=on  OutDataTypeStr=Inherit: Same as input  ParamDataTypeStr=Inherit: Same as input
  Sum1 : Sum  Inputs=|+-+  SaturateOnIntegerOverflow=on
  Sum2 : Sum  Inputs=|+---  SaturateOnIntegerOverflow=on
  sqrt(3) : Gain  SaturateOnIntegerOverflow=on  OutDataTypeStr=Inherit: Same as input  ParamDataTypeStr=Inherit: Same as input
  id : Outport
  iq : Outport  Port=2
  phase : Outport  Port=3
  u : Outport  Port=4
  wires:
  Integrator/1 -> Mux/7, phase/1
  w/1 -> Product2/2, Integrator/1, Product1/3, Product/3  "w"
  Mux/1 -> Fcn/1, Fcn1/1, u/1
  Fcn/1 -> Sum1/1  "ud"
  Sum1/1 -> 1/Ld/1
  1/Ld/1 -> Integrator1/1
  Integrator1/1 -> Rd/1, id/1, Product1/2  "id"
  Rd/1 -> Sum1/2  "R*id"
  Fcn1/1 -> Sum2/1  "uq"
  Sum2/1 -> 1/Lq/1
  1/Lq/1 -> Integrator2/1
  Integrator2/1 -> Rq/1, iq/1, Product/2  "iq"
  Rq/1 -> Sum2/2  "R*iq"
  Product/1 -> Sum1/3  "w*iq*Lq"
  Product1/1 -> Sum2/3  "w*id*Ld"
  Product2/1 -> sqrt(3)/1
  psi/1 -> Product2/1
  Lq/1 -> Product/1
  Ld/1 -> Product1/1
  ud/1 -> Mux/1
  ua/1 -> Mux/2
  ue/1 -> Mux/3
  ub/1 -> Mux/4
  uf/1 -> Mux/5
  uc/1 -> Mux/6
  sqrt(3)/1 -> Sum2/4  "sqrt(3)*w*psi"

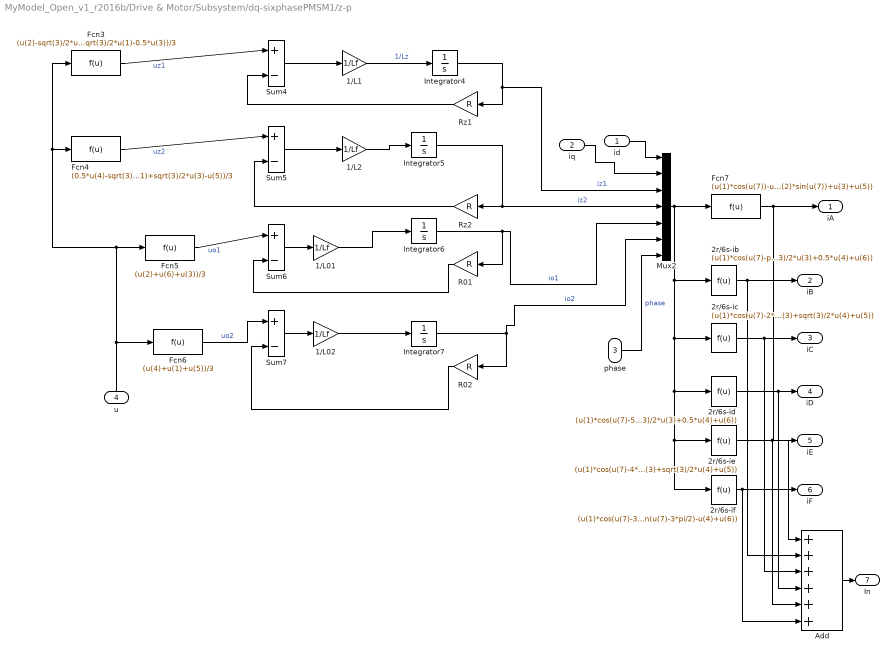
== system MyModel_Open_v1_r2016b/Drive & Motor/Subsystem/dq-sixphasePMSM1/z-p ==
  id : Inport
  iq : Inport  Port=2
  phase : Inport  Port=3
  u : Inport  Port=4
  1/L01 : Gain  Gain=1/Lf  SaturateOnIntegerOverflow=on  OutDataTypeStr=Inherit: Same as input  ParamDataTypeStr=Inherit: Same as input
  1/L02 : Gain  Gain=1/Lf  SaturateOnIntegerOverflow=on  OutDataTypeStr=Inherit: Same as input  ParamDataTypeStr=Inherit: Same as input
  1/L1 : Gain  Gain=1/Lf  SaturateOnIntegerOverflow=on  OutDataTypeStr=Inherit: Same as input  ParamDataTypeStr=Inherit: Same as input
  1/L2 : Gain  Gain=1/Lf  SaturateOnIntegerOverflow=on  OutDataTypeStr=Inherit: Same as input  ParamDataTypeStr=Inherit: Same as input
  2r/6s-ib : Fcn  Expr=(u(1)*cos(u(7)-pi/6)-u(2)*sin(u(7)-pi/6)-sqrt(3)/2*u(3)+0.5*u(4)+u(6))
  2r/6s-ic : Fcn  Expr=(u(1)*cos(u(7)-2*pi/3)-u(2)*sin(u(7)-2*pi/3)-0.5*u(3)+sqrt(3)/2*u(4)+u(5))
  2r/6s-id : Fcn  Expr=(u(1)*cos(u(7)-5*pi/6)-u(2)*sin(u(7)-5*pi/6)+sqrt(3)/2*u(3)+0.5*u(4)+u(6))
  2r/6s-ie : Fcn  Expr=(u(1)*cos(u(7)-4*pi/3)-u(2)*sin(u(7)-4*pi/3)-0.5*u(3)+sqrt(3)/2*u(4)+u(5))
  2r/6s-if : Fcn  Expr=(u(1)*cos(u(7)-3*pi/2)-u(2)*sin(u(7)-3*pi/2)-u(4)+u(6))
  Add : Sum  Inputs=++++++
  Fcn3 : Fcn  Expr=(u(2)-sqrt(3)/2*u(4)-0.5*u(6)+sqrt(3)/2*u(1)-0.5*u(3))/3
  Fcn4 : Fcn  Expr=(0.5*u(4)-sqrt(3)/2*u(6)+0.5*u(1)+sqrt(3)/2*u(3)-u(5))/3
  Fcn5 : Fcn  Expr=(u(2)+u(6)+u(3))/3
  Fcn6 : Fcn  Expr=(u(4)+u(1)+u(5))/3
  Fcn7 : Fcn  Expr=(u(1)*cos(u(7))-u(2)*sin(u(7))+u(3)+u(5))
  Integrator{4..7} (4 alike) : Integrator
  Mux2 : Mux  Inputs=7
  R01 : Gain  Gain=R  SaturateOnIntegerOverflow=on  OutDataTypeStr=Inherit: Same as input  ParamDataTypeStr=Inherit: Same as input
  R02 : Gain  Gain=R  SaturateOnIntegerOverflow=on  OutDataTypeStr=Inherit: Same as input  ParamDataTypeStr=Inherit: Same as input
  Rz1 : Gain  Gain=R  SaturateOnIntegerOverflow=on  OutDataTypeStr=Inherit: Same as input  ParamDataTypeStr=Inherit: Same as input
  Rz2 : Gain  Gain=R  SaturateOnIntegerOverflow=on  OutDataTypeStr=Inherit: Same as input  ParamDataTypeStr=Inherit: Same as input
  Sum{4..7} (4 alike) : Sum  Inputs=|+-  SaturateOnIntegerOverflow=on
  iA : Outport
  iB : Outport  Port=2
  iC : Outport  Port=3
  iD : Outport  Port=4
  iE : Outport  Port=5
  iF : Outport  Port=6
  In : Outport  Port=7
  wires:
  Mux2/1 -> Fcn7/1, 2r/6s-ic/1, 2r/6s-id/1, 2r/6s-ie/1, 2r/6s-if/1, 2r/6s-ib/1
  R02/1 -> Sum7/2
  R01/1 -> Sum6/2
  Rz2/1 -> Sum5/2
  Rz1/1 -> Sum4/2
  Integrator7/1 -> Mux2/6, R02/1  "io2"
  1/L02/1 -> Integrator7/1
  Sum7/1 -> 1/L02/1
  Integrator6/1 -> R01/1, Mux2/5  "io1"
  1/L01/1 -> Integrator6/1
  Sum6/1 -> 1/L01/1
  id/1 -> Mux2/1
  iq/1 -> Mux2/2
  u/1 -> Fcn4/1, Fcn3/1, Fcn5/1, Fcn6/1
  phase/1 -> Mux2/7  "phase"
  Fcn7/1 -> Add/1, iA/1
  2r/6s-ib/1 -> Add/2, iB/1
  2r/6s-id/1 -> Add/4, iD/1
  2r/6s-ie/1 -> Add/5, iE/1
  2r/6s-if/1 -> Add/6, iF/1
  1/L2/1 -> Integrator5/1
  Sum5/1 -> 1/L2/1
  Fcn6/1 -> Sum7/1  "uo2"
  Fcn5/1 -> Sum6/1  "uo1"
  Integrator4/1 -> Rz1/1, Mux2/3  "iz1"
  Integrator5/1 -> Mux2/4, Rz2/1  "iz2"
  Fcn3/1 -> Sum4/1  "uz1"
  Fcn4/1 -> Sum5/1  "uz2"
  Add/1 -> In/1
  2r/6s-ic/1 -> Add/3, iC/1
  Sum4/1 -> 1/L1/1
  1/L1/1 -> Integrator4/1  "1/Lz"

== matlab function MyModel_Open_v1_r2016b/Drive & Motor/Embedded MATLAB Function ==
  data: uo output; uab input; ua output; ubc input; ucd input; ude input; uef input; ub output; uc output; ud output; ue output; uf output
function [uo,ua,ub,uc,ud,ue,uf] = fcn(uab,ubc,ucd,ude,uef)

%#codegen
uxx = [uab,ubc,ucd,ude,uef,0,0]';
T = [0 1 -1 0 0 0 0;
     0 0 1 -1 0 0 0;
     1 0 0 1 -1 0 0;
     0 0 0 0 1 -1 0;
     0 0 0 0 0 1 -1;
     0 1 1 1 0 0 0;
     0 0 0 0 1 1 1];
I = T \ uxx;
uo = I(1);
ua = I(2);
ub = I(3);
uc = I(4);
ud = I(5);
ue = I(6);
uf = I(7);

== matlab function MyModel_Open_v1_r2016b/Drive & Motor/Embedded MATLAB Function1 ==
  data: uo output; uab input; ua output; ubc input; ucd input; ude input; uef input; ub output; uc output; ud output; ue output; uf output
function [uo,ua,ub,uc,ud,ue,uf] = fcn(uab,ubc,ucd,ude,uef)

%#codegen
uxx = [uab,ubc,ucd,ude,uef,0,0]';
T = [0 1 -1 0 0 0 0;
     0 0 1 -1 0 0 0;
     1 0 0 1 -1 0 0;
     0 0 0 0 1 -1 0;
     0 0 0 0 0 1 -1;
     0 1 1 1 0 0 0;
     0 0 0 0 1 1 1];
I = T \ uxx;
uo = I(1);
ua = I(2);
ub = I(3);
uc = I(4);
ud = I(5);
ue = I(6);
uf = I(7);

== matlab function MyModel_Open_v1_r2016b/Drive & Motor/clark1 ==
  data: falpha output; fa input; fbeta output; fb input; fc input; fd input; fe input; fx output; fy output; fo1 output; fo2 output; ff input
function [falpha,fbeta,fx,fy,fo1,fo2] = clark(fa,fb,fc,fd,fe,ff)

T=1/3*[1,  (-1/2),    (-1/2),       sqrt(3)/2,  -sqrt(3)/2,  0;
       0,  sqrt(3)/2, (-sqrt(3)/2), 1/2,        1/2,        -1;
       1,  (-1/2),    (-1/2),       -sqrt(3)/2, sqrt(3)/2,   0;
       0,  -sqrt(3)/2,sqrt(3)/2,    1/2,        1/2,        -1;
       1,  1,         1,            0,          0,           0;
       0,  0,         0,            1,          1,           1];
X=[fa;fb;fc;fd;fe;ff];
Y=T*X;
falpha=Y(1);
fbeta=Y(2);
fx=Y(3);
fy=Y(4);
fo1=Y(5);
fo2=Y(6);
end

== matlab function MyModel_Open_v1_r2016b/SVPWM2/Embedded MATLAB Function1 ==
  data: N input; t1 output; Ualpha input; Ubeta input; Tpwm input; t2 output; t3 output; t4 output; t0 output; udc input; Ux input; Uy input; t1cp output; t2cp output; t3cp output; t4cp output
function [t1, t2, t3, t4, t0, t1cp, t2cp, t3cp, t4cp] = fcn(N, Ualpha, Ubeta, Tpwm, udc, Ux,Uy)

m=sqrt(3)/2+1/2*1i;

%等幅clarke反变换
ab44=1/3*udc*[1,m^4,m^8,m,m^5,m^9]*[1;0;0;1;0;0];
xy44=1/3*udc*[1,m^8,m^4,m^5,m,m^9]*[1;0;0;1;0;0];

ab64=1/3*udc*[1,m^4,m^8,m,m^5,m^9]*[1;1;0;1;0;0];
xy64=1/3*udc*[1,m^8,m^4,m^5,m,m^9]*[1;1;0;1;0;0];
        
ab66=1/3*udc*[1,m^4,m^8,m,m^5,m^9]*[1;1;0;1;1;0];
xy66=1/3*udc*[1,m^8,m^4,m^5,m,m^9]*[1;1;0;1;1;0];

ab26=1/3*udc*[1,m^4,m^8,m,m^5,m^9]*[0;1;0;1;1;0];
xy26=1/3*udc*[1,m^8,m^4,m^5,m,m^9]*[0;1;0;1;1;0];

ab22=1/3*udc*[1,m^4,m^8,m,m^5,m^9]*[0;1;0;0;1;0];
xy22=1/3*udc*[1,m^8,m^4,m^5,m,m^9]*[0;1;0;0;1;0];

ab32=1/3*udc*[1,m^4,m^8,m,m^5,m^9]*[0;1;1;0;1;0];
xy32=1/3*udc*[1,m^8,m^4,m^5,m,m^9]*[0;1;1;0;1;0];

ab33=1/3*udc*[1,m^4,m^8,m,m^5,m^9]*[0;1;1;0;1;1];
xy33=1/3*udc*[1,m^8,m^4,m^5,m,m^9]*[0;1;1;0;1;1];

ab13=1/3*udc*[1,m^4,m^8,m,m^5,m^9]*[0;0;1;0;1;1];
xy13=1/3*udc*[1,m^8,m^4,m^5,m,m^9]*[0;0;1;0;1;1];

ab11=1/3*udc*[1,m^4,m^8,m,m^5,m^9]*[0;0;1;0;0;1];
xy11=1/3*udc*[1,m^8,m^4,m^5,m,m^9]*[0;0;1;0;0;1];

ab51=1/3*udc*[1,m^4,m^8,m,m^5,m^9]*[1;0;1;0;0;1];
xy51=1/3*udc*[1,m^8,m^4,m^5,m,m^9]*[1;0;1;0;0;1];

ab55=1/3*udc*[1,m^4,m^8,m,m^5,m^9]*[1;0;1;1;0;1];
xy55=1/3*udc*[1,m^8,m^4,m^5,m,m^9]*[1;0;1;1;0;1];

ab45=1/3*udc*[1,m^4,m^8,m,m^5,m^9]*[1;0;0;1;0;1];
xy45=1/3*udc*[1,m^8,m^4,m^5,m,m^9]*[1;0;0;1;0;1];

switch N
    case 1
        X=[real(ab55),real(ab45),real(ab44),real(ab64);
           imag(ab55),imag(ab45),imag(ab44),imag(ab64);
           real(xy55),real(xy45),real(xy44),real(xy64);
           imag(xy55),imag(xy45),imag(xy44),imag(xy64)];

    case 2
        X=[real(ab45),real(ab44),real(ab64),real(ab66);
           imag(ab45),imag(ab44),imag(ab64),imag(ab66);
           real(xy45),real(xy44),real(xy64),real(xy66);
           imag(xy45),imag(xy44),imag(xy64),imag(xy66)];

    case 3
        X=[real(ab44),real(ab64),real(ab66),real(ab26);
           imag(ab44),imag(ab64),imag(ab66),imag(ab26);
           real(xy44),real(xy64),real(xy66),real(xy26);
           imag(xy44),imag(xy64),imag(xy66),imag(xy26)];

    case 4
        X=[real(ab64),real(ab66),real(ab26),real(ab22);
           imag(ab64),imag(ab66),imag(ab26),imag(ab22);
           real(xy64),real(xy66),real(xy26),real(xy22);
           imag(xy64),imag(xy66),imag(xy26),imag(xy22)];

    case 5
        X=[real(ab66),real(ab26),real(ab22),real(ab32);
           imag(ab66),imag(ab26),imag(ab22),imag(ab32);
           real(xy66),real(xy26),real(xy22),real(xy32);
           imag(xy66),imag(xy26),imag(xy22),imag(xy32)];

    case 6
        X=[real(ab26),real(ab22),real(ab32),real(ab33);
           imag(ab26),imag(ab22),imag(ab32),imag(ab33);
           real(xy26),real(xy22),real(xy32),real(xy33);
           imag(xy26),imag(xy22),imag(xy32),imag(xy33)];

    case 7
        X=[real(ab22),real(ab32),real(ab33),real(ab13);
           imag(ab22),imag(ab32),imag(ab33),imag(ab13);
           real(xy22),real(xy32),real(xy33),real(xy13);
           imag(xy22),imag(xy32),imag(xy33),imag(xy13)];

    case 8
        X=[real(ab32),real(ab33),real(ab13),real(ab11);
           imag(ab32),imag(ab33),imag(ab13),imag(ab11);
           real(xy32),real(xy33),real(xy13),real(xy11);
           imag(xy32),imag(xy33),imag(xy13),imag(xy11)];

    case 9
        X=[real(ab33),real(ab13),real(ab11),real(ab51);
           imag(ab33),imag(ab13),imag(ab11),imag(ab51);
           real(xy33),real(xy13),real(xy11),real(xy51);
           imag(xy33),imag(xy13),imag(xy11),imag(xy51)];

    case 10
        X=[real(ab13),real(ab11),real(ab51),real(ab55);
           imag(ab13),imag(ab11),imag(ab51),imag(ab55);
           real(xy13),real(xy11),real(xy51),real(xy55);
           imag(xy13),imag(xy11),imag(xy51),imag(xy55)];

    case 11
        X=[real(ab11),real(ab51),real(ab55),real(ab45);
           imag(ab11),imag(ab51),imag(ab55),imag(ab45);
           real(xy11),real(xy51),real(xy55),real(xy45);
           imag(xy11),imag(xy51),imag(xy55),imag(xy45)];

    case 12
        X=[real(ab51),real(ab55),real(ab45),real(ab44);
           imag(ab51),imag(ab55),imag(ab45),imag(ab44);
           real(xy51),real(xy55),real(xy45),real(xy44);
           imag(xy51),imag(xy55),imag(xy45),imag(xy44)];

    otherwise
        X=[0,0,0,0;
           0,0,0,0;
           0,0,0,0;
           0,0,0,0];

end
Y=[Ualpha;Ubeta;Ux;Uy]*Tpwm;
T = X \ Y;

% t1=T(1);
% if t1<15e-6
%     t1=15e-6;
% end
% t2=T(2);
% if t2<15e-6
%     t2=15e-6;
% end
% t3=T(3);
% if t3<1e-6
%     t3=1e-6;
% end
% t4=T(4);
% if t4<1e-6
%     t4=1e-6;
% end

t1=T(1);
t2=T(2);
t3=T(3);
t4=T(4);
t1cp = 0;
t2cp = 0;
t3cp = 0;
t4cp = 0;
% if T(1) >= 0
%     t1 = T(1);
% else
%     t1 = 0;
%     t1cp = -T(1);
% end
% if T(2) >= 0
%     t2 = T(2);
% else
%     t2 = 0;
%     t2cp = -T(2);
% end
% if T(3) >= 0
%     t3 = T(3);
% else
%     t3 = 0;
%     t3cp = -T(3);
% end
% if T(4) >= 0
%     t4 = T(4);
% else
%     t4 = 0;
%     t4cp = -T(4);
% end

Tsum=t1+t2+t3+t4;
if Tsum>Tpwm
    t1=t1*Tpwm/Tsum;
    t2=t2*Tpwm/Tsum;
    t3=t3*Tpwm/Tsum;
    t4=t4*Tpwm/Tsum;
end
t0=Tpwm-t1-t2-t3-t4;
end
